simulink model "generatorlosowej"  (R2022a)
settings: Solver=VariableStepAuto  StartTime=0.0  StopTime=300  RelTol=1e-3
settings Model: Creator=M  LastModifiedBy=M

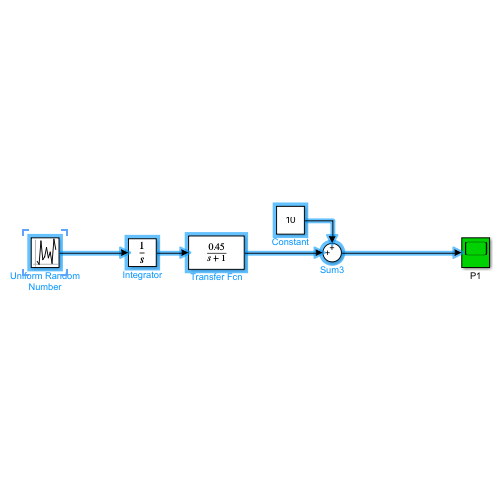
[thumbnail: Simulink's stored preview of the top-level diagram]
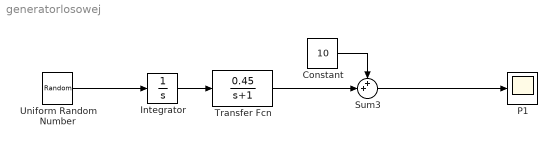
== system generatorlosowej ==
  Constant : Constant  Value=10
  Integrator : Integrator
  P1 : Scope
  Sum3 : Sum  Inputs=++|
  Transfer Fcn : TransferFcn  Numerator=[0.45]  Denominator=[1 1]
  Uniform Random Number : UniformRandomNumber  Seed=65165  SampleTime=0.1
  wires:
  Transfer Fcn/1 -> Sum3/2
  Sum3/1 -> P1/1
  Constant/1 -> Sum3/1
  Uniform Random Number/1 -> Integrator/1
  Integrator/1 -> Transfer Fcn/1
